simulink model "tip_interaction"  (R2016b)
settings: Solver=VariableStepAuto  StartTime=0.0  StopTime=.0000005  RelTol=1e-3
values from neighbouring files (symbols this model uses):
  u0 = -0*scl    (= 0)    [force_sim.m]
undefined symbols (not defined in the file or in its folder): params
settings Model: Creator=arnold  LastModifiedBy=arnold

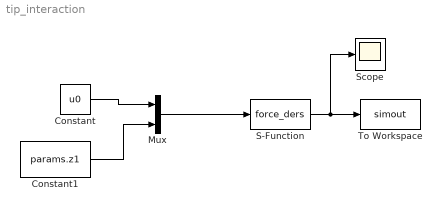
== system tip_interaction ==
  Constant : Constant  Value=u0
  Constant1 : Constant  Value=params.z1
  Mux : Mux  Inputs=2
  S-Function : S-Function  FunctionName=force_ders  Parameters=params  SFunctionDeploymentMode=off  EnableBusSupport=off
  Scope : Scope
  To Workspace : ToWorkspace  VariableName=simout  SaveFormat=Timeseries  SampleTime=-1
  wires:
  Constant/1 -> Mux/1
  Constant1/1 -> Mux/2
  Mux/1 -> S-Function/1
  S-Function/1 -> Scope/1, To Workspace/1
